simulink model "gpkfPathOpt_th"  (R2020a)
settings: Solver=FixedStepAuto  StartTime=0.0  StopTime=algFinTime*60  FixedStep=hiLvlCtrl.kfgpTimeStep*60/2  RelTol=1e-3
values from neighbouring files (symbols this model uses):
  mpckfgp = GP.KalmanFilteredGaussianProcess(spaceKernel,timeKernel,     'windPowerLaw',altitudes,mpckfgpTimeStep)    [matlabTestkfgp.m]
undefined symbols (not defined in the file or in its folder): hiLvlCtrl
libraries: simulink x1, gpkfPathOpt_cl x1
settings Model: Creator=Ayaz  LastModifiedBy=Ayaz

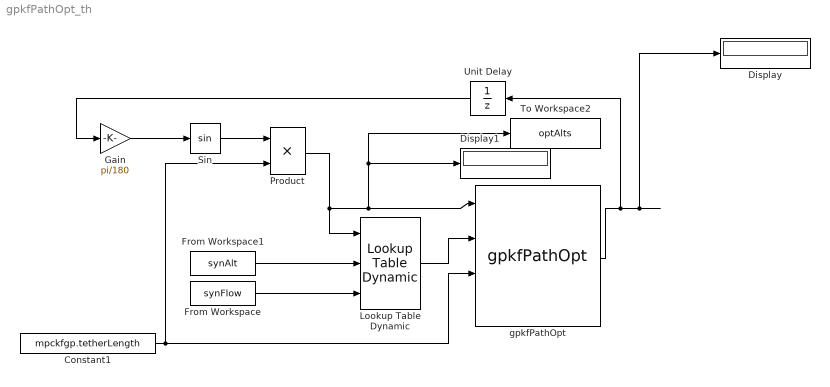
== system gpkfPathOpt_th ==
  Constant1 : Constant  Value=mpckfgp.tetherLength
  Display : Display
  Display1 : Display
  From Workspace : FromWorkspace  VariableName=synFlow
  From Workspace1 : FromWorkspace  VariableName=synAlt
  Gain : Gain  Gain=pi/180
  Lookup Table Dynamic : simulink/Lookup Tables/Lookup Table Dynamic  LookUpMeth=Interpolation-Use End Values  OutDataType=fixdt('double')  OutScaling=[]  OutputDataTypeScalingMode=Specify via dialog  OutDataTypeStr=double  DoSatur=off
  Product : Product
  Sin : Trigonometry
  To Workspace2 : ToWorkspace  VariableName=optAlts  SaveFormat=Timeseries  SampleTime=-1
  Unit Delay : UnitDelay  InitialCondition=hiLvlCtrl.initVals  SampleTime=-1  HasFrameUpgradeWarning=on
  gpkfPathOpt : gpkfPathOpt_cl/gpkfPathOpt  hiLvlCtrl=hiLvlCtrl
  wires:
  From Workspace1/1 -> Lookup Table Dynamic/2
  From Workspace/1 -> Lookup Table Dynamic/3
  Product/1 -> Lookup Table Dynamic/1, To Workspace2/1, Display1/1, gpkfPathOpt/1
  Lookup Table Dynamic/1 -> gpkfPathOpt/2
  Constant1/1 -> Product/2, gpkfPathOpt/3
  Gain/1 -> Sin/1
  Sin/1 -> Product/1
  gpkfPathOpt/1 -> Unit Delay/1, Display/1
  Unit Delay/1 -> Gain/1
